simulink model "chap6_4sim"  (Simulink 7.7)
settings: Solver=ode45  StartTime=0.0  StopTime=2  FixedStep=0.001  RelTol=1e-3
settings Model: Creator=ljk  LastModifiedBy=ljk  ExtModeTrigMode=oneshot  ExtModeArmWhenConnect=off
settings DataIOCC: LimitDataPoints=off  SignalLoggingName=sigsOut
settings OptimizationCC: BooleanDataType=off
settings DebuggingCC: SaveWithParameterizedLinksMsg=none  SignalResolutionControl=TryResolveAllWithWarning  SolverPrmCheckMsg=none  MultiTaskDSMMsg=warning  MultiTaskCondExecSysMsg=none  StrictBusMsg=None
settings HardwareCC: TargetUnknown=on
settings RTWCC: IncludeERTFirstTime=on

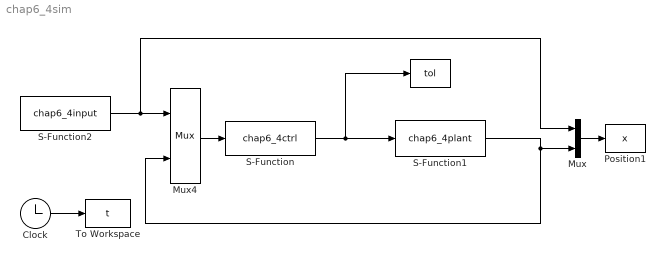
== system chap6_4sim ==
  "  " : ToWorkspace  VariableName=tol  SampleTime=-1  SaveFormat=Array
  Clock : Clock
      settings: Decimation=10
  Mux : Mux  Inputs=2
  Mux4 : Mux  Inputs=2
  Position1 : ToWorkspace  VariableName=x  SampleTime=-1  SaveFormat=Array
  S-Function : S-Function  FunctionName=chap6_4ctrl  EnableBusSupport=off
  S-Function1 : S-Function  FunctionName=chap6_4plant  EnableBusSupport=off
  S-Function2 : S-Function  FunctionName=chap6_4input  EnableBusSupport=off
  To Workspace : ToWorkspace  VariableName=t  SampleTime=-1  SaveFormat=Array
  wires:
  S-Function/1 -> S-Function1/1, "  "/1
  S-Function1/1 -> Mux4/2, Mux/2
  Clock/1 -> To Workspace/1
  Mux4/1 -> S-Function/1
  S-Function2/1 -> Mux4/1, Mux/1
  Mux/1 -> Position1/1
